simulink model "controllo_giunti_2"  (R2020b)
settings: Solver=FixedStepAuto  StartTime=0.0  StopTime=1  FixedStep=0.001  RelTol=1e-3
libraries: robotcorelib x1
(part 1 of 2)
settings Model: Creator=frasi  LastModifiedBy=frasi

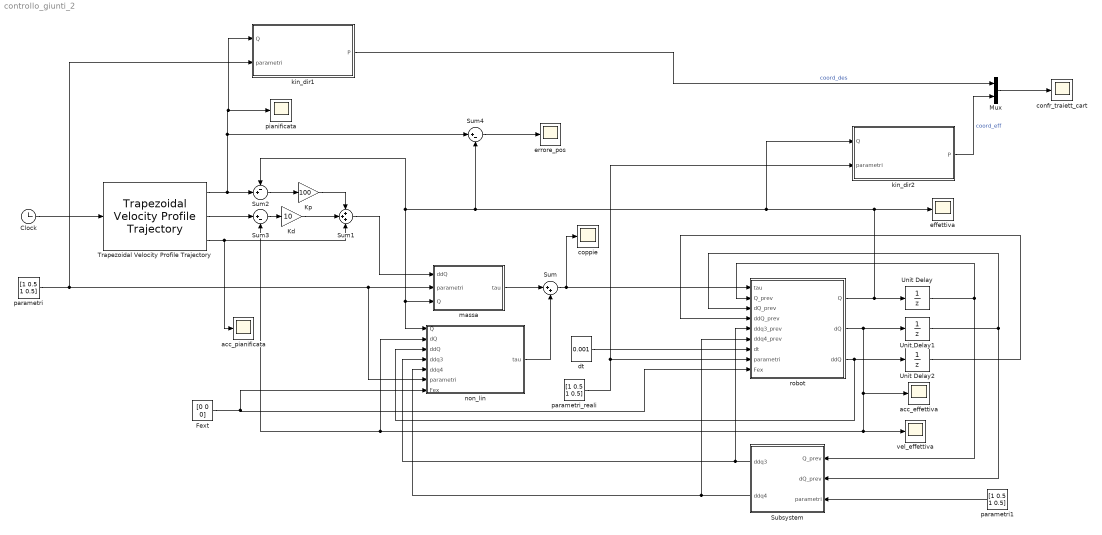
== system controllo_giunti_2 ==
  Clock : Clock
  Fext : Constant  Value=[0 0 0]
  Kd : Gain  Gain=10
  Kp : Gain  Gain=100
  Mux : Mux  Inputs=2
  Subsystem : Subsystem
  Sum : Sum  Inputs=|++
  Sum1 : Sum  Inputs=+++
  Sum2 : Sum  Inputs=-+|
  Sum3 : Sum  Inputs=|+-
  Sum4 : Sum  Inputs=|+-
  Trapezoidal Velocity Profile Trajectory : robotcorelib/Trapezoidal Velocity Profile Trajectory  WaypointSource=Internal  Waypoints=[0.5 0.7; 0.7 0.5; pi/4 pi/3]  NumParams=1  Parameter1=End Time  Parameter2=End Time  ParameterSource=Internal  PeakVelocity=[ 2; 2 ]  Acceleration=[ 1; 2 ]  EndTime=[ 1; 1 ;1]  AccelTime=[ 1; 2 ]  SimulateUsing=Interpreted execution
      settings: SourceProductBaseCode=NV,RO,RR,UV
  Unit Delay : UnitDelay  InitialCondition=[0.5 0.7 pi/4]  SampleTime=-1  HasFrameUpgradeWarning=on
  Unit Delay1 : UnitDelay  InitialCondition=[0 0 0]  SampleTime=-1  HasFrameUpgradeWarning=on
  Unit Delay2 : UnitDelay  InitialCondition=[0 0 0]  SampleTime=-1  HasFrameUpgradeWarning=on
  acc_effettiva : Scope
  acc_pianificata : Scope
  confr_traiett_cart : Scope
  coppie : Scope
  dt : Constant  Value=0.001
  effettiva : Scope
  errore_pos : Scope
  kin_dir1 : MATLAB Function  TreatAsAtomicUnit=on
  kin_dir2 : MATLAB Function  TreatAsAtomicUnit=on
  massa : MATLAB Function  TreatAsAtomicUnit=on
  non_lin : MATLAB Function  TreatAsAtomicUnit=on
  parametri : Constant  Value=[1 0.5 1 0.5]
  parametri1 : Constant  Value=[1 0.5 1 0.5]
  parametri_reali : Constant  Value=[1 0.5 1 0.5]
  pianificata : Scope
  robot : MATLAB Function  TreatAsAtomicUnit=on
  vel_effettiva : Scope
  wires:
  Clock/1 -> Trapezoidal Velocity Profile Trajectory/1
  parametri/1 -> kin_dir1/2(parametri), non_lin/6(parametri), massa/2(parametri)
  massa/1(tau) -> Sum/1
  dt/1 -> robot/7(dt)
  robot/1(Q) -> Unit Delay/1, Sum4/2, Sum2/1, massa/3(Q), non_lin/1(Q), kin_dir2/1(Q), effettiva/1
  robot/2(dQ) -> Unit Delay1/1, non_lin/2(dQ), Sum3/2, vel_effettiva/1, acc_effettiva/1
  Unit Delay/1 -> Subsystem/1(Q_prev), robot/2(Q_prev)
  Unit Delay1/1 -> Subsystem/2(dQ_prev), robot/3(dQ_prev)
  Sum/1 -> coppie/1, robot/1(tau)
  Sum1/1 -> massa/1(ddQ)
  Trapezoidal Velocity Profile Trajectory/2 -> Sum3/1
  Sum2/1 -> Kp/1
  Sum3/1 -> Kd/1
  Kp/1 -> Sum1/1
  Kd/1 -> Sum1/2
  Trapezoidal Velocity Profile Trajectory/3 -> acc_pianificata/1, Sum1/3
  non_lin/1(tau) -> Sum/2
  Trapezoidal Velocity Profile Trajectory/1 -> Sum4/1, kin_dir1/1(Q), pianificata/1, Sum2/2
  robot/3(ddQ) -> non_lin/3(ddQ), Unit Delay2/1
  parametri_reali/1 -> kin_dir2/2(parametri), robot/8(parametri)
  Sum4/1 -> errore_pos/1
  kin_dir1/1(P) -> Mux/1  "coord_des"
  kin_dir2/1(P) -> Mux/2  "coord_eff"
  Mux/1 -> confr_traiett_cart/1
  Fext/1 -> non_lin/7(Fex), robot/9(Fex)
  parametri1/1 -> Subsystem/3(parametri)
  Subsystem/2(ddq4) -> non_lin/5(ddq4), robot/6(ddq4_prev)
  Unit Delay2/1 -> robot/4(ddQ_prev)
  Subsystem/1(ddq3) -> non_lin/4(ddq3), robot/5(ddq3_prev)

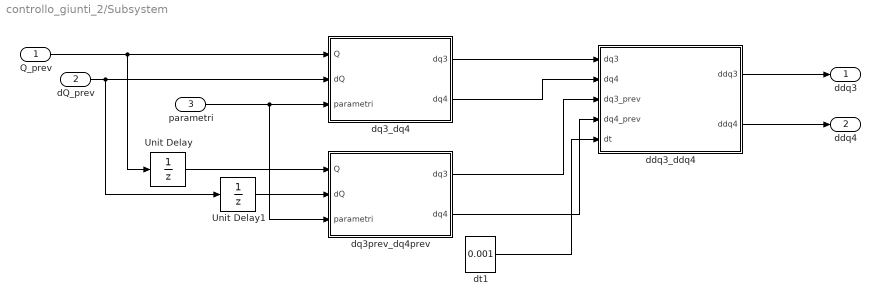
== system controllo_giunti_2/Subsystem ==
  Q_prev : Inport
  dQ_prev : Inport  Port=2
  parametri : Inport  Port=3
  Unit Delay : UnitDelay  InitialCondition=[0.5 0.7 pi/4]  SampleTime=-1  HasFrameUpgradeWarning=on
  Unit Delay1 : UnitDelay  InitialCondition=[0 0 0]  SampleTime=-1  HasFrameUpgradeWarning=on
  ddq3_ddq4 : MATLAB Function  TreatAsAtomicUnit=on
  dq3_dq4 : MATLAB Function  TreatAsAtomicUnit=on
  dq3prev_dq4prev : MATLAB Function  TreatAsAtomicUnit=on
  dt1 : Constant  Value=0.001
  ddq3 : Outport
  ddq4 : Outport  Port=2
  wires:
  ddq3_ddq4/1(ddq3) -> ddq3/1
  parametri/1 -> dq3prev_dq4prev/3(parametri), dq3_dq4/3(parametri)
  Q_prev/1 -> Unit Delay/1, dq3_dq4/1(Q)
  dq3_dq4/2(dq4) -> ddq3_ddq4/2(dq4)
  ddq3_ddq4/2(ddq4) -> ddq4/1
  dq3_dq4/1(dq3) -> ddq3_ddq4/1(dq3)
  dt1/1 -> ddq3_ddq4/5(dt)
  dq3prev_dq4prev/1(dq3) -> ddq3_ddq4/3(dq3_prev)
  dq3prev_dq4prev/2(dq4) -> ddq3_ddq4/4(dq4_prev)
  dQ_prev/1 -> Unit Delay1/1, dq3_dq4/2(dQ)
  Unit Delay1/1 -> dq3prev_dq4prev/2(dQ)
  Unit Delay/1 -> dq3prev_dq4prev/1(Q)

== matlab function controllo_giunti_2/non_lin ==
  data: Q input; tau output; dQ input; ddQ input; ddq3 input; ddq4 input; parametri input; Fex input
function tau = non_lin(Q,dQ,ddQ,ddq3,ddq4,parametri,Fex)
l=parametri(1);
d=parametri(2);
m1=parametri(3);
ma=parametri(4);

xc1=Q(1);
xc5=Q(2);
q2=Q(3);

dxc1=dQ(1);
dxc5=dQ(2);
dq2=dQ(3);

ddxc1=ddQ(1);
ddxc5=ddQ(2);
ddq2=ddQ(3);

Fx=Fex(1);
Fy=Fex(2);
Mf=Fex(3);

I2 = ma*l^2/4 + 1/12 *ma*l^2;
I5 = I2;
I3 = I2 + 1/12 * ma*d^2 + ma*(d^2/4+l^2/4);

q3 = ...
 -q2 - 2*atan((2*l*xc5 + (-(2*l*xc1 + l^2 + l^2*tan(q2/2)^2 + xc1^2 + xc5^2 + xc1^2*tan(q2/2)^2 + xc5^2*tan(q2/2)^2 - 4*l*xc5*tan(q2/2) - 2*l*xc1*tan(q2/2)^2)*(2*l*xc1 - 3*l^2 - 3*l^2*tan(q2/2)^2 + xc1^2 + xc5^2 + xc1^2*tan(q2/2)^2 + xc5^2*tan(q2/2)^2 - 4*l*xc5*tan(q2/2) - 2*l*xc1*tan(q2/2)^2))^(1/2) - 4*l^2*tan(q2/2) + 2*l*xc5*tan(q2/2)^2)/(3*l^2*tan(q2/2)^2 - l^2 + xc1^2 + xc5^2 + xc1^2*tan(q2/2)^2 + xc5^2*tan(q2/2)^2 - 4*l*xc5*tan(q2/2) - 4*l*xc1*tan(q2/2)^2) - (4*(l*xc5 - 2*l^2*tan(q2/2) + l*xc5*tan(q2/2)^2))/(3*l^2*tan(q2/2)^2 - l^2 + xc1^2 + xc5^2 + xc1^2*tan(q2/2)^2 + xc5^2*tan(q2/2)^2 - 4*l*xc5*tan(q2/2) - 4*l*xc1*tan(q2/2)^2));
q4 = ...
2*atan((2*l*xc5 + (-(2*l*xc1 + l^2 + l^2*tan(q2/2)^2 + xc1^2 + xc5^2 + xc1^2*tan(q2/2)^2 + xc5^2*tan(q2/2)^2 - 4*l*xc5*tan(q2/2) - 2*l*xc1*tan(q2/2)^2)*(2*l*xc1 - 3*l^2 - 3*l^2*tan(q2/2)^2 + xc1^2 + xc5^2 + xc1^2*tan(q2/2)^2 + xc5^2*tan(q2/2)^2 - 4*l*xc5*tan(q2/2) - 2*l*xc1*tan(q2/2)^2))^(1/2) - 4*l^2*tan(q2/2) + 2*l*xc5*tan(q2/2)^2)/(3*l^2*tan(q2/2)^2 - l^2 + xc1^2 + xc5^2 + xc1^2*tan(q2/2)^2 + xc5^2*tan(q2/2)^2 - 4*l*xc5*tan(q2/2) - 4*l*xc1*tan(q2/2)^2)) + 2*atan((2*l*xc5 + (-(2*l*xc1 + l^2 + l^2*tan(q2/2)^2 + xc1^2 + xc5^2 + xc1^2*tan(q2/2)^2 + xc5^2*tan(q2/2)^2 - 4*l*xc5*tan(q2/2) - 2*l*xc1*tan(q2/2)^2)*(2*l*xc1 - 3*l^2 - 3*l^2*tan(q2/2)^2 + xc1^2 + xc5^2 + xc1^2*tan(q2/2)^2 + xc5^2*tan(q2/2)^2 - 4*l*xc5*tan(q2/2) - 2*l*xc1*tan(q2/2)^2))^(1/2) - 4*l^2*tan(q2/2) + 2*l*xc5*tan(q2/2)^2)/(3*l^2*tan(q2/2)^2 - l^2 + xc1^2 + xc5^2 + xc1^2*tan(q2/2)^2 + xc5^2*tan(q2/2)^2 - 4*l*xc5*tan(q2/2) - 4*l*xc1*tan(q2/2)^2) - (4*(l*xc5 - 2*l^2*tan(q2/2) + l*xc5*tan(q2/2)^2))/(3*l^2*tan(q2/2)^2 - l^2 + xc1^2 + xc5^2 + xc1^2*tan(q2/2)^2 + xc5^2*tan(q2/2)^2 - 4*l*xc5*tan(q2/2) - 4*l*xc1*tan(q2/2)^2));

dq3 =...
(2*dxc5*((2*l + (4*sin(q2)*l^3 - 4*sin(2*q2)*l^2*xc1 - 4*cos(2*q2)*l^2*xc5 - 4*sin(q2)*l*xc1^2 + 8*cos(q2)*l*xc1*xc5 - 12*sin(q2)*l*xc5^2 + 4*xc1^2*xc5 + 4*xc5^3)/(2*(3*l^4 + 4*cos(q2)*l^3*xc1 - 4*sin(q2)*l^3*xc5 - 2*cos(2*q2)*l^2*xc1^2 + 4*sin(2*q2)*l^2*xc1*xc5 + 2*cos(2*q2)*l^2*xc5^2 - 4*cos(q2)*l*xc1^3 + 4*sin(q2)*l*xc1^2*xc5 - 4*cos(q2)*l*xc1*xc5^2 + 4*sin(q2)*l*xc5^3 - xc1^4 - 2*xc1^2*xc5^2 - xc5^4)^(1/2)))/(l^2 - 2*l*xc1 + xc1^2 + xc5^2 - 2*l^2*cos(q2) + 2*l*xc1*cos(q2) - 2*l*xc5*sin(q2)) + ((2*xc5 - 2*l*sin(q2))*(2*l^2*sin(q2) + (3*l^4 + 4*cos(q2)*l^3*xc1 - 4*sin(q2)*l^3*xc5 - 2*cos(2*q2)*l^2*xc1^2 + 4*sin(2*q2)*l^2*xc1*xc5 + 2*cos(2*q2)*l^2*xc5^2 - 4*cos(q2)*l*xc1^3 + 4*sin(q2)*l*xc1^2*xc5 - 4*cos(q2)*l*xc1*xc5^2 + 4*sin(q2)*l*xc5^3 - xc1^4 - 2*xc1^2*xc5^2 - xc5^4)^(1/2) - 2*l*xc5))/(l^2 - 2*l*xc1 + xc1^2 + xc5^2 - 2*l^2*cos(q2) + 2*l*xc1*cos(q2) - 2*l*xc5*sin(q2))^2))/((2*l^2*sin(q2) + (3*l^4 + 4*cos(q2)*l^3*xc1 - 4*sin(q2)*l^3*xc5 - 2*cos(2*q2)*l^2*xc1^2 + 4*sin(2*q2)*l^2*xc1*xc5 + 2*cos(2*q2)*l^2*xc5^2 - 4*cos(q2)*l*xc1^3 + 4*sin(q2)*l*xc1^2*xc5 - 4*cos(q2)*l*xc1*xc5^2 + 4*sin(q2)*l*xc5^3 - xc1^4 - 2*xc1^2*xc5^2 - xc5^4)^(1/2) - 2*l*xc5)^2/(l^2 - 2*l*xc1 + xc1^2 + xc5^2 - 2*l^2*cos(q2) + 2*l*xc1*cos(q2) - 2*l*xc5*sin(q2))^2 + 1) - dq2*((2*(((- 4*sin(q2)*l^3*xc1 - 4*cos(q2)*l^3*xc5 + 4*sin(2*q2)*l^2*xc1^2 + 8*cos(2*q2)*l^2*xc1*xc5 - 4*sin(2*q2)*l^2*xc5^2 + 4*sin(q2)*l*xc1^3 + 4*cos(q2)*l*xc1^2*xc5 + 4*sin(q2)*l*xc1*xc5^2 + 4*cos(q2)*l*xc5^3)/(2*(3*l^4 + 4*cos(q2)*l^3*xc1 - 4*sin(q2)*l^3*xc5 - 2*cos(2*q2)*l^2*xc1^2 + 4*sin(2*q2)*l^2*xc1*xc5 + 2*cos(2*q2)*l^2*xc5^2 - 4*cos(q2)*l*xc1^3 + 4*sin(q2)*l*xc1^2*xc5 - 4*cos(q2)*l*xc1*xc5^2 + 4*sin(q2)*l*xc5^3 - xc1^4 - 2*xc1^2*xc5^2 - xc5^4)^(1/2)) + 2*l^2*cos(q2))/(l^2 - 2*l*xc1 + xc1^2 + xc5^2 - 2*l^2*cos(q2) + 2*l*xc1*cos(q2) - 2*l*xc5*sin(q2)) + ((2*l*xc5*cos(q2) - 2*l^2*sin(q2) + 2*l*xc1*sin(q2))*(2*l^2*sin(q2) + (3*l^4 + 4*cos(q2)*l^3*xc1 - 4*sin(q2)*l^3*xc5 - 2*cos(2*q2)*l^2*xc1^2 + 4*sin(2*q2)*l^2*xc1*xc5 + 2*cos(2*q2)*l^2*xc5^2 - 4*cos(q2)*l*xc1^3 + 4*sin(q2)*l*xc1^2*xc5 - 4*cos(q2)*l*xc1*xc5^2 + 4*sin(q2)*l*xc5^3 - xc1^4 - 2*xc1^2*xc5^2 - xc5^4)^(1/2) - 2*l*xc5))/(l^2 - 2*l*xc1 + xc1^2 + xc5^2 - 2*l^2*cos(q2) + 2*l*xc1*cos(q2) - 2*l*xc5*sin(q2))^2))/((2*l^2*sin(q2) + (3*l^4 + 4*cos(q2)*l^3*xc1 - 4*sin(q2)*l^3*xc5 - 2*cos(2*q2)*l^2*xc1^2 + 4*sin(2*q2)*l^2*xc1*xc5 + 2*cos(2*q2)*l^2*xc5^2 - 4*cos(q2)*l*xc1^3 + 4*sin(q2)*l*xc1^2*xc5 - 4*cos(q2)*l*xc1*xc5^2 + 4*sin(q2)*l*xc5^3 - xc1^4 - 2*xc1^2*xc5^2 - xc5^4)^(1/2) - 2*l*xc5)^2/(l^2 - 2*l*xc1 + xc1^2 + xc5^2 - 2*l^2*cos(q2) + 2*l*xc1*cos(q2) - 2*l*xc5*sin(q2))^2 + 1) + 1) + (2*dxc1*(((2*xc1 - 2*l + 2*l*cos(q2))*(2*l^2*sin(q2) + (3*l^4 + 4*cos(q2)*l^3*xc1 - 4*sin(q2)*l^3*xc5 - 2*cos(2*q2)*l^2*xc1^2 + 4*sin(2*q2)*l^2*xc1*xc5 + 2*cos(2*q2)*l^2*xc5^2 - 4*cos(q2)*l*xc1^3 + 4*sin(q2)*l*xc1^2*xc5 - 4*cos(q2)*l*xc1*xc5^2 + 4*sin(q2)*l*xc5^3 - xc1^4 - 2*xc1^2*xc5^2 - xc5^4)^(1/2) - 2*l*xc5))/(l^2 - 2*l*xc1 + xc1^2 + xc5^2 - 2*l^2*cos(q2) + 2*l*xc1*cos(q2) - 2*l*xc5*sin(q2))^2 + (- 4*cos(q2)*l^3 + 4*cos(2*q2)*l^2*xc1 - 4*sin(2*q2)*l^2*xc5 + 12*cos(q2)*l*xc1^2 - 8*sin(q2)*l*xc1*xc5 + 4*cos(q2)*l*xc5^2 + 4*xc1^3 + 4*xc1*xc5^2)/(2*(l^2 - 2*l*xc1 + xc1^2 + xc5^2 - 2*l^2*cos(q2) + 2*l*xc1*cos(q2) - 2*l*xc5*sin(q2))*(3*l^4 + 4*cos(q2)*l^3*xc1 - 4*sin(q2)*l^3*xc5 - 2*cos(2*q2)*l^2*xc1^2 + 4*sin(2*q2)*l^2*xc1*xc5 + 2*cos(2*q2)*l^2*xc5^2 - 4*cos(q2)*l*xc1^3 + 4*sin(q2)*l*xc1^2*xc5 - 4*cos(q2)*l*xc1*xc5^2 + 4*sin(q2)*l*xc5^3 - xc1^4 - 2*xc1^2*xc5^2 - xc5^4)^(1/2))))/((2*l^2*sin(q2) + (3*l^4 + 4*cos(q2)*l^3*xc1 - 4*sin(q2)*l^3*xc5 - 2*cos(2*q2)*l^2*xc1^2 + 4*sin(2*q2)*l^2*xc1*xc5 + 2*cos(2*q2)*l^2*xc5^2 - 4*cos(q2)*l*xc1^3 + 4*sin(q2)*l*xc1^2*xc5 - 4*cos(q2)*l*xc1*xc5^2 + 4*sin(q2)*l*xc5^3 - xc1^4 - 2*xc1^2*xc5^2 - xc5^4)^(1/2) - 2*l*xc5)^2/(l^2 - 2*l*xc1 + xc1^2 + xc5^2 - 2*l^2*cos(q2) + 2*l*xc1*cos(q2) - 2*l*xc5*sin(q2))^2 + 1);

dq4 =...
 - dxc1*((2*(((2*xc1 - 2*l + 2*l*cos(q2))*((3*l^4 + 4*cos(q2)*l^3*xc1 - 4*sin(q2)*l^3*xc5 - 2*cos(2*q2)*l^2*xc1^2 + 4*sin(2*q2)*l^2*xc1*xc5 + 2*cos(2*q2)*l^2*xc5^2 - 4*cos(q2)*l*xc1^3 + 4*sin(q2)*l*xc1^2*xc5 - 4*cos(q2)*l*xc1*xc5^2 + 4*sin(q2)*l*xc5^3 - xc1^4 - 2*xc1^2*xc5^2 - xc5^4)^(1/2) - 2*l^2*sin(q2) + 2*l*xc5))/(l^2 - 2*l*xc1 + xc1^2 + xc5^2 - 2*l^2*cos(q2) + 2*l*xc1*cos(q2) - 2*l*xc5*sin(q2))^2 + (2*(xc1 + l*cos(q2))*(- l^2 + 2*cos(q2)*l*xc1 - 2*sin(q2)*l*xc5 + xc1^2 + xc5^2))/((l^2 - 2*l*xc1 + xc1^2 + xc5^2 - 2*l^2*cos(q2) + 2*l*xc1*cos(q2) - 2*l*xc5*sin(q2))*(3*l^4 + 4*cos(q2)*l^3*xc1 - 4*sin(q2)*l^3*xc5 - 2*cos(2*q2)*l^2*xc1^2 + 4*sin(2*q2)*l^2*xc1*xc5 + 2*cos(2*q2)*l^2*xc5^2 - 4*cos(q2)*l*xc1^3 + 4*sin(q2)*l*xc1^2*xc5 - 4*cos(q2)*l*xc1*xc5^2 + 4*sin(q2)*l*xc5^3 - xc1^4 - 2*xc1^2*xc5^2 - xc5^4)^(1/2))))/(((3*l^4 + 4*cos(q2)*l^3*xc1 - 4*sin(q2)*l^3*xc5 - 2*cos(2*q2)*l^2*xc1^2 + 4*sin(2*q2)*l^2*xc1*xc5 + 2*cos(2*q2)*l^2*xc5^2 - 4*cos(q2)*l*xc1^3 + 4*sin(q2)*l*xc1^2*xc5 - 4*cos(q2)*l*xc1*xc5^2 + 4*sin(q2)*l*xc5^3 - xc1^4 - 2*xc1^2*xc5^2 - xc5^4)^(1/2) - 2*l^2*sin(q2) + 2*l*xc5)^2/(l^2 - 2*l*xc1 + xc1^2 + xc5^2 - 2*l^2*cos(q2) + 2*l*xc1*cos(q2) - 2*l*xc5*sin(q2))^2 + 1) + (2*(((2*xc1 - 2*l + 2*l*cos(q2))*(2*l^2*sin(q2) + (3*l^4 + 4*cos(q2)*l^3*xc1 - 4*sin(q2)*l^3*xc5 - 2*cos(2*q2)*l^2*xc1^2 + 4*sin(2*q2)*l^2*xc1*xc5 + 2*cos(2*q2)*l^2*xc5^2 - 4*cos(q2)*l*xc1^3 + 4*sin(q2)*l*xc1^2*xc5 - 4*cos(q2)*l*xc1*xc5^2 + 4*sin(q2)*l*xc5^3 - xc1^4 - 2*xc1^2*xc5^2 - xc5^4)^(1/2) - 2*l*xc5))/(l^2 - 2*l*xc1 + xc1^2 + xc5^2 - 2*l^2*cos(q2) + 2*l*xc1*cos(q2) - 2*l*xc5*sin(q2))^2 + (2*(xc1 + l*cos(q2))*(- l^2 + 2*cos(q2)*l*xc1 - 2*sin(q2)*l*xc5 + xc1^2 + xc5^2))/((l^2 - 2*l*xc1 + xc1^2 + xc5^2 - 2*l^2*cos(q2) + 2*l*xc1*cos(q2) - 2*l*xc5*sin(q2))*(3*l^4 + 4*cos(q2)*l^3*xc1 - 4*sin(q2)*l^3*xc5 - 2*cos(2*q2)*l^2*xc1^2 + 4*sin(2*q2)*l^2*xc1*xc5 + 2*cos(2*q2)*l^2*xc5^2 - 4*cos(q2)*l*xc1^3 + 4*sin(q2)*l*xc1^2*xc5 - 4*cos(q2)*l*xc1*xc5^2 + 4*sin(q2)*l*xc5^3 - xc1^4 - 2*xc1^2*xc5^2 - xc5^4)^(1/2))))/((2*l^2*sin(q2) + (3*l^4 + 4*cos(q2)*l^3*xc1 - 4*sin(q2)*l^3*xc5 - 2*cos(2*q2)*l^2*xc1^2 + 4*sin(2*q2)*l^2*xc1*xc5 + 2*cos(2*q2)*l^2*xc5^2 - 4*cos(q2)*l*xc1^3 + 4*sin(q2)*l*xc1^2*xc5 - 4*cos(q2)*l*xc1*xc5^2 + 4*sin(q2)*l*xc5^3 - xc1^4 - 2*xc1^2*xc5^2 - xc5^4)^(1/2) - 2*l*xc5)^2/(l^2 - 2*l*xc1 + xc1^2 + xc5^2 - 2*l^2*cos(q2) + 2*l*xc1*cos(q2) - 2*l*xc5*sin(q2))^2 + 1)) - dxc5*((2*((2*l + (2*sin(q2)*l^3 - 2*sin(2*q2)*l^2*xc1 - 2*cos(2*q2)*l^2*xc5 - 2*sin(q2)*l*xc1^2 + 4*cos(q2)*l*xc1*xc5 - 6*sin(q2)*l*xc5^2 + 2*xc1^2*xc5 + 2*xc5^3)/(3*l^4 + 4*cos(q2)*l^3*xc1 - 4*sin(q2)*l^3*xc5 - 2*cos(2*q2)*l^2*xc1^2 + 4*sin(2*q2)*l^2*xc1*xc5 + 2*cos(2*q2)*l^2*xc5^2 - 4*cos(q2)*l*xc1^3 + 4*sin(q2)*l*xc1^2*xc5 - 4*cos(q2)*l*xc1*xc5^2 + 4*sin(q2)*l*xc5^3 - xc1^4 - 2*xc1^2*xc5^2 - xc5^4)^(1/2))/(l^2 - 2*l*xc1 + xc1^2 + xc5^2 - 2*l^2*cos(q2) + 2*l*xc1*cos(q2) - 2*l*xc5*sin(q2)) + ((2*xc5 - 2*l*sin(q2))*(2*l^2*sin(q2) + (3*l^4 + 4*cos(q2)*l^3*xc1 - 4*sin(q2)*l^3*xc5 - 2*cos(2*q2)*l^2*xc1^2 + 4*sin(2*q2)*l^2*xc1*xc5 + 2*cos(2*q2)*l^2*xc5^2 - 4*cos(q2)*l*xc1^3 + 4*sin(q2)*l*xc1^2*xc5 - 4*cos(q2)*l*xc1*xc5^2 + 4*sin(q2)*l*xc5^3 - xc1^4 - 2*xc1^2*xc5^2 - xc5^4)^(1/2) - 2*l*xc5))/(l^2 - 2*l*xc1 + xc1^2 + xc5^2 - 2*l^2*cos(q2) + 2*l*xc1*cos(q2) - 2*l*xc5*sin(q2))^2))/((2*l^2*sin(q2) + (3*l^4 + 4*cos(q2)*l^3*xc1 - 4*sin(q2)*l^3*xc5 - 2*cos(2*q2)*l^2*xc1^2 + 4*sin(2*q2)*l^2*xc1*xc5 + 2*cos(2*q2)*l^2*xc5^2 - 4*cos(q2)*l*xc1^3 + 4*sin(q2)*l*xc1^2*xc5 - 4*cos(q2)*l*xc1*xc5^2 + 4*sin(q2)*l*xc5^3 - xc1^4 - 2*xc1^2*xc5^2 - xc5^4)^(1/2) - 2*l*xc5)^2/(l^2 - 2*l*xc1 + xc1^2 + xc5^2 - 2*l^2*cos(q2) + 2*l*xc1*cos(q2) - 2*l*xc5*sin(q2))^2 + 1) - (2*((2*l - (2*sin(q2)*l^3 - 2*sin(2*q2)*l^2*xc1 - 2*cos(2*q2)*l^2*xc5 - 2*sin(q2)*l*xc1^2 + 4*cos(q2)*l*xc1*xc5 - 6*sin(q2)*l*xc5^2 + 2*xc1^2*xc5 + 2*xc5^3)/(3*l^4 + 4*cos(q2)*l^3*xc1 - 4*sin(q2)*l^3*xc5 - 2*cos(2*q2)*l^2*xc1^2 + 4*sin(2*q2)*l^2*xc1*xc5 + 2*cos(2*q2)*l^2*xc5^2 - 4*cos(q2)*l*xc1^3 + 4*sin(q2)*l*xc1^2*xc5 - 4*cos(q2)*l*xc1*xc5^2 + 4*sin(q2)*l*xc5^3 - xc1^4 - 2*xc1^2*xc5^2 - xc5^4)^(1/2))/(l^2 - 2*l*xc1 + xc1^2 + xc5^2 - 2*l^2*cos(q2) + 2*l*xc1*cos(q2) - 2*l*xc5*sin(q2)) - ((2*xc5 - 2*l*sin(q2))*((3*l^4 + 4*cos(q2)*l^3*xc1 - 4*sin(q2)*l^3*xc5 - 2*cos(2*q2)*l^2*xc1^2 + 4*sin(2*q2)*l^2*xc1*xc5 + 2*cos(2*q2)*l^2*xc5^2 - 4*cos(q2)*l*xc1^3 + 4*sin(q2)*l*xc1^2*xc5 - 4*cos(q2)*l*xc1*xc5^2 + 4*sin(q2)*l*xc5^3 - xc1^4 - 2*xc1^2*xc5^2 - xc5^4)^(1/2) - 2*l^2*sin(q2) + 2*l*xc5))/(l^2 - 2*l*xc1 + xc1^2 + xc5^2 - 2*l^2*cos(q2) + 2*l*xc1*cos(q2) - 2*l*xc5*sin(q2))^2))/(((3*l^4 + 4*cos(q2)*l^3*xc1 - 4*sin(q2)*l^3*xc5 - 2*cos(2*q2)*l^2*xc1^2 + 4*sin(2*q2)*l^2*xc1*xc5 + 2*cos(2*q2)*l^2*xc5^2 - 4*cos(q2)*l*xc1^3 + 4*sin(q2)*l*xc1^2*xc5 - 4*cos(q2)*l*xc1*xc5^2 + 4*sin(q2)*l*xc5^3 - xc1^4 - 2*xc1^2*xc5^2 - xc5^4)^(1/2) - 2*l^2*sin(q2) + 2*l*xc5)^2/(l^2 - 2*l*xc1 + xc1^2 + xc5^2 - 2*l^2*cos(q2) + 2*l*xc1*cos(q2) - 2*l*xc5*sin(q2))^2 + 1)) - dq2*((2*((2*l^2*cos(q2) - (2*l*(- sin(q2)*l^2*xc1 - cos(q2)*l^2*xc5 + sin(2*q2)*l*xc1^2 + 2*cos(2*q2)*l*xc1*xc5 - sin(2*q2)*l*xc5^2 + sin(q2)*xc1^3 + cos(q2)*xc1^2*xc5 + sin(q2)*xc1*xc5^2 + cos(q2)*xc5^3))/(3*l^4 + 4*cos(q2)*l^3*xc1 - 4*sin(q2)*l^3*xc5 - 2*cos(2*q2)*l^2*xc1^2 + 4*sin(2*q2)*l^2*xc1*xc5 + 2*cos(2*q2)*l^2*xc5^2 - 4*cos(q2)*l*xc1^3 + 4*sin(q2)*l*xc1^2*xc5 - 4*cos(q2)*l*xc1*xc5^2 + 4*sin(q2)*l*xc5^3 - xc1^4 - 2*xc1^2*xc5^2 - xc5^4)^(1/2))/(l^2 - 2*l*xc1 + xc1^2 + xc5^2 - 2*l^2*cos(q2) + 2*l*xc1*cos(q2) - 2*l*xc5*sin(q2)) - (2*l*(xc5*cos(q2) - l*sin(q2) + xc1*sin(q2))*((3*l^4 + 4*cos(q2)*l^3*xc1 - 4*sin(q2)*l^3*xc5 - 2*cos(2*q2)*l^2*xc1^2 + 4*sin(2*q2)*l^2*xc1*xc5 + 2*cos(2*q2)*l^2*xc5^2 - 4*cos(q2)*l*xc1^3 + 4*sin(q2)*l*xc1^2*xc5 - 4*cos(q2)*l*xc1*xc5^2 + 4*sin(q2)*l*xc5^3 - xc1^4 - 2*xc1^2*xc5^2 - xc5^4)^(1/2) - 2*l^2*sin(q2) + 2*l*xc5))/(l^2 - 2*l*xc1 + xc1^2 + xc5^2 - 2*l^2*cos(q2) + 2*l*xc1*cos(q2) - 2*l*xc5*sin(q2))^2))/(((3*l^4 + 4*cos(q2)*l^3*xc1 - 4*sin(q2)*l^3*xc5 - 2*cos(2*q2)*l^2*xc1^2 + 4*sin(2*q2)*l^2*xc1*xc5 + 2*cos(2*q2)*l^2*xc5^2 - 4*cos(q2)*l*xc1^3 + 4*sin(q2)*l*xc1^2*xc5 - 4*cos(q2)*l*xc1*xc5^2 + 4*sin(q2)*l*xc5^3 - xc1^4 - 2*xc1^2*xc5^2 - xc5^4)^(1/2) - 2*l^2*sin(q2) + 2*l*xc5)^2/(l^2 - 2*l*xc1 + xc1^2 + xc5^2 - 2*l^2*cos(q2) + 2*l*xc1*cos(q2) - 2*l*xc5*sin(q2))^2 + 1) - (2*((2*l^2*cos(q2) + (2*l*(- sin(q2)*l^2*xc1 - cos(q2)*l^2*xc5 + sin(2*q2)*l*xc1^2 + 2*cos(2*q2)*l*xc1*xc5 - sin(2*q2)*l*xc5^2 + sin(q2)*xc1^3 + cos(q2)*xc1^2*xc5 + sin(q2)*xc1*xc5^2 + cos(q2)*xc5^3))/(3*l^4 + 4*cos(q2)*l^3*xc1 - 4*sin(q2)*l^3*xc5 - 2*cos(2*q2)*l^2*xc1^2 + 4*sin(2*q2)*l^2*xc1*xc5 + 2*cos(2*q2)*l^2*xc5^2 - 4*cos(q2)*l*xc1^3 + 4*sin(q2)*l*xc1^2*xc5 - 4*cos(q2)*l*xc1*xc5^2 + 4*sin(q2)*l*xc5^3 - xc1^4 - 2*xc1^2*xc5^2 - xc5^4)^(1/2))/(l^2 - 2*l*xc1 + xc1^2 + xc5^2 - 2*l^2*cos(q2) + 2*l*xc1*cos(q2) - 2*l*xc5*sin(q2)) + (2*l*(xc5*cos(q2) - l*sin(q2) + xc1*sin(q2))*(2*l^2*sin(q2) + (3*l^4 + 4*cos(q2)*l^3*xc1 - 4*sin(q2)*l^3*xc5 - 2*cos(2*q2)*l^2*xc1^2 + 4*sin(2*q2)*l^2*xc1*xc5 + 2*cos(2*q2)*l^2*xc5^2 - 4*cos(q2)*l*xc1^3 + 4*sin(q2)*l*xc1^2*xc5 - 4*cos(q2)*l*xc1*xc5^2 + 4*sin(q2)*l*xc5^3 - xc1^4 - 2*xc1^2*xc5^2 - xc5^4)^(1/2) - 2*l*xc5))/(l^2 - 2*l*xc1 + xc1^2 + xc5^2 - 2*l^2*cos(q2) + 2*l*xc1*cos(q2) - 2*l*xc5*sin(q2))^2))/((2*l^2*sin(q2) + (3*l^4 + 4*cos(q2)*l^3*xc1 - 4*sin(q2)*l^3*xc5 - 2*cos(2*q2)*l^2*xc1^2 + 4*sin(2*q2)*l^2*xc1*xc5 + 2*cos(2*q2)*l^2*xc5^2 - 4*cos(q2)*l*xc1^3 + 4*sin(q2)*l*xc1^2*xc5 - 4*cos(q2)*l*xc1*xc5^2 + 4*sin(q2)*l*xc5^3 - xc1^4 - 2*xc1^2*xc5^2 - xc5^4)^(1/2) - 2*l*xc5)^2/(l^2 - 2*l*xc1 + xc1^2 + xc5^2 - 2*l^2*cos(q2) + 2*l*xc1*cos(q2) - 2*l*xc5*sin(q2))^2 + 1));

ddx2=ddxc1-l/2*(cos(q2)*dq2^2+sin(q2)*ddq2);
q5=q2+q3+q4-pi;
dq5=dq2+dq3+dq4;
ddq5=ddq2+ddq3+ddq4;
ddy4=ddxc5+ddq5*l/2*cos(q5)-dq5^2*l/2*sin(q5);

g=9.81;

G=...
[                  -(ma*(3*l*cos(q4) + 3*l*cos(2*q2 + 2*q3 + q4) - d*sin(q4) + d*sin(2*q2 + 2*q3 + q4)))/(4*l*sin(q4));...
(d*ma*cos(q4) - d*ma*cos(2*q2 + 2*q3 + q4) + 4*l*m1*sin(q4) + 5*l*ma*sin(q4) + 3*l*ma*sin(2*q2 + 2*q3 + q4))/(4*l*sin(q4));...
-(ma*(3*l*sin(q2 + 2*q3 + q4) - d*cos(q2 + 2*q3 + q4) - 6*l*sin(q2 + q4) + d*cos(q2 - q4) + 3*l*sin(q2 - q4)))/(4*sin(q4))];

V=...
   [(4*Mf*cos(q2 + q3 + q4) + 3*l*ma*cos(q4) + 3*l*ma*cos(2*q2 + 2*q3 + q4) - d*ma*sin(q4) + d*ma*sin(2*q2 + 2*q3 + q4) - 4*I3*ddq3*cos(q2 + q3 + q4) + 4*I5*ddq3*cos(q2 + q3) + 4*I5*ddq4*cos(q2 + q3) - 4*Fx*l*sin(q4) - 4*dq2^2*l^2*ma*sin(q2 + q4) + 2*ddq3*l^2*ma*cos(q2 + q3 + q4) + 4*dq2^2*l^2*ma*sin(q2 - q4) - 2*ddq3*l^2*ma*cos(q2 + q3 - q4) - 3*g*l*ma*cos(q4) - 3*g*l*ma*cos(2*q2 + 2*q3 + q4) + d*g*ma*sin(q4) - d*g*ma*sin(2*q2 + 2*q3 + q4) + 4*ddx2*l*ma*sin(q4) - 2*dq2^2*l^2*ma*sin(q2 + q3 + q4) - 2*dq3^2*l^2*ma*sin(q2 + q3 + q4) + 2*dq2^2*l^2*ma*sin(q2 + q3 - q4) + 2*dq3^2*l^2*ma*sin(q2 + q3 - q4) + 4*d*ddq3*l*ma*sin(q2 + q3 + q4) + 4*d*dq2^2*l*ma*cos(q2 + q3 + q4) + 4*d*dq3^2*l*ma*cos(q2 + q3 + q4) - 4*d*ddq3*l*ma*sin(q2 + q3 - q4) - 4*dq2*dq3*l^2*ma*sin(q2 + q3 + q4) - 4*d*dq2^2*l*ma*cos(q2 + q3 - q4) - 4*d*dq3^2*l*ma*cos(q2 + q3 - q4) + 4*dq2*dq3*l^2*ma*sin(q2 + q3 - q4) + 8*d*dq2*dq3*l*ma*cos(q2 + q3 + q4) - 8*d*dq2*dq3*l*ma*cos(q2 + q3 - q4))/(4*l*sin(q4));...
                                                                                                                                                                                                                                                                                                                                                                                                                                                                                                                                                                                                                            -(4*Mf*sin(q2 + q3 + q4) + d*ma*cos(q4) - d*ma*cos(2*q2 + 2*q3 + q4) + 4*l*m1*sin(q4) + 5*l*ma*sin(q4) + 3*l*ma*sin(2*q2 + 2*q3 + q4) - 4*I3*ddq3*sin(q2 + q3 + q4) + 4*I5*ddq3*sin(q2 + q3) + 4*I5*ddq4*sin(q2 + q3) - d*g*ma*cos(q4) + d*g*ma*cos(2*q2 + 2*q3 + q4) - 4*ddy4*l*ma*sin(q4) - 4*g*l*m1*sin(q4) - 5*g*l*ma*sin(q4) - 3*g*l*ma*sin(2*q2 + 2*q3 + q4))/(4*l*sin(q4));...
                                                       (4*Mf*sin(q3 + q4) + 2*Fx*l*cos(q2 - q4) + 2*Fy*l*sin(q2 - q4) + d*ma*cos(q2 - q4) + 3*l*ma*sin(q2 - q4) - d*ma*cos(q2 + 2*q3 + q4) - 2*Fx*l*cos(q2 + q4) + 3*l*ma*sin(q2 + 2*q3 + q4) - 4*I3*ddq3*sin(q3 + q4) - 2*Fy*l*sin(q2 + q4) - 6*l*ma*sin(q2 + q4) + 4*I5*ddq3*sin(q3) + 4*I5*ddq4*sin(q3) + 2*dq2^2*l^2*ma*cos(q3 + q4) + 2*dq3^2*l^2*ma*cos(q3 + q4) + d*g*ma*cos(q2 + 2*q3 + q4) - 2*ddq3*l^2*ma*sin(q3 - q4) - 3*g*l*ma*sin(q2 + 2*q3 + q4) + 6*g*l*ma*sin(q2 + q4) - 2*dq2^2*l^2*ma*cos(q3 - q4) - 2*dq3^2*l^2*ma*cos(q3 - q4) - d*g*ma*cos(q2 - q4) + 2*ddq3*l^2*ma*sin(q3 + q4) - 3*g*l*ma*sin(q2 - q4) + 4*d*ddq3*l*ma*cos(q3 - q4) + 4*dq2*dq3*l^2*ma*cos(q3 + q4) + 4*d*dq2^2*l*ma*sin(q3 + q4) + 4*d*dq3^2*l*ma*sin(q3 + q4) - 4*dq2*dq3*l^2*ma*cos(q3 - q4) - 4*d*dq2^2*l*ma*sin(q3 - q4) - 4*d*dq3^2*l*ma*sin(q3 - q4) - 4*d*ddq3*l*ma*cos(q3 + q4) + 8*d*dq2*dq3*l*ma*sin(q3 + q4) - 8*d*dq2*dq3*l*ma*sin(q3 - q4))/(4*sin(q4))];
N=G+V;

tau=N;
end

== matlab function controllo_giunti_2/massa ==
  data: ddQ input; parametri input; tau output; Q input
function tau = massa(ddQ,parametri,Q)
l=parametri(1);
d=parametri(2);
m1=parametri(3);
ma=parametri(4);

xc1=Q(1);
xc5=Q(2);
q2=Q(3);

q3 = ...
 -q2 - 2*atan((2*l*xc5 + (-(2*l*xc1 + l^2 + l^2*tan(q2/2)^2 + xc1^2 + xc5^2 + xc1^2*tan(q2/2)^2 + xc5^2*tan(q2/2)^2 - 4*l*xc5*tan(q2/2) - 2*l*xc1*tan(q2/2)^2)*(2*l*xc1 - 3*l^2 - 3*l^2*tan(q2/2)^2 + xc1^2 + xc5^2 + xc1^2*tan(q2/2)^2 + xc5^2*tan(q2/2)^2 - 4*l*xc5*tan(q2/2) - 2*l*xc1*tan(q2/2)^2))^(1/2) - 4*l^2*tan(q2/2) + 2*l*xc5*tan(q2/2)^2)/(3*l^2*tan(q2/2)^2 - l^2 + xc1^2 + xc5^2 + xc1^2*tan(q2/2)^2 + xc5^2*tan(q2/2)^2 - 4*l*xc5*tan(q2/2) - 4*l*xc1*tan(q2/2)^2) - (4*(l*xc5 - 2*l^2*tan(q2/2) + l*xc5*tan(q2/2)^2))/(3*l^2*tan(q2/2)^2 - l^2 + xc1^2 + xc5^2 + xc1^2*tan(q2/2)^2 + xc5^2*tan(q2/2)^2 - 4*l*xc5*tan(q2/2) - 4*l*xc1*tan(q2/2)^2));
q4 = ...
2*atan((2*l*xc5 + (-(2*l*xc1 + l^2 + l^2*tan(q2/2)^2 + xc1^2 + xc5^2 + xc1^2*tan(q2/2)^2 + xc5^2*tan(q2/2)^2 - 4*l*xc5*tan(q2/2) - 2*l*xc1*tan(q2/2)^2)*(2*l*xc1 - 3*l^2 - 3*l^2*tan(q2/2)^2 + xc1^2 + xc5^2 + xc1^2*tan(q2/2)^2 + xc5^2*tan(q2/2)^2 - 4*l*xc5*tan(q2/2) - 2*l*xc1*tan(q2/2)^2))^(1/2) - 4*l^2*tan(q2/2) + 2*l*xc5*tan(q2/2)^2)/(3*l^2*tan(q2/2)^2 - l^2 + xc1^2 + xc5^2 + xc1^2*tan(q2/2)^2 + xc5^2*tan(q2/2)^2 - 4*l*xc5*tan(q2/2) - 4*l*xc1*tan(q2/2)^2)) + 2*atan((2*l*xc5 + (-(2*l*xc1 + l^2 + l^2*tan(q2/2)^2 + xc1^2 + xc5^2 + xc1^2*tan(q2/2)^2 + xc5^2*tan(q2/2)^2 - 4*l*xc5*tan(q2/2) - 2*l*xc1*tan(q2/2)^2)*(2*l*xc1 - 3*l^2 - 3*l^2*tan(q2/2)^2 + xc1^2 + xc5^2 + xc1^2*tan(q2/2)^2 + xc5^2*tan(q2/2)^2 - 4*l*xc5*tan(q2/2) - 2*l*xc1*tan(q2/2)^2))^(1/2) - 4*l^2*tan(q2/2) + 2*l*xc5*tan(q2/2)^2)/(3*l^2*tan(q2/2)^2 - l^2 + xc1^2 + xc5^2 + xc1^2*tan(q2/2)^2 + xc5^2*tan(q2/2)^2 - 4*l*xc5*tan(q2/2) - 4*l*xc1*tan(q2/2)^2) - (4*(l*xc5 - 2*l^2*tan(q2/2) + l*xc5*tan(q2/2)^2))/(3*l^2*tan(q2/2)^2 - l^2 + xc1^2 + xc5^2 + xc1^2*tan(q2/2)^2 + xc5^2*tan(q2/2)^2 - 4*l*xc5*tan(q2/2) - 4*l*xc1*tan(q2/2)^2));


I2 = ma*l^2/4 + 1/12 *ma*l^2;
I5 = I2;
I3 = I2 + 1/12 * ma*d^2 + ma*(d^2/4+l^2/4);

M =...
[      m1 + 2*ma,  0,                                        (I5*cos(q2 + q3) - I3*cos(q2 + q3 + q4))/(l*sin(q4)) - ma*(l*sin(q2 + q3) - 2*d*cos(q2 + q3) + 2*l*sin(q2));...
              0, m1,                                                                                              -(I5*sin(q2 + q3) - I3*sin(q2 + q3 + q4))/(l*sin(q4));...
-2*l*ma*sin(q2),  0, (I2*sin(q4) + I5*sin(q3) - I3*cos(q3)*sin(q4) - I3*cos(q4)*sin(q3) + 2*l^2*ma*sin(q4) + l^2*ma*cos(q3)*sin(q4) + 2*d*l*ma*sin(q3)*sin(q4))/sin(q4)];
 
tau=M*ddQ;
end

== matlab function controllo_giunti_2/robot ==
  data: tau input; Q output; Q_prev input; dQ_prev input; ddQ_prev input; ddq3_prev input; ddq4_prev input; dt input; parametri input; dQ output; ddQ output; Fex input
function [Q,dQ,ddQ] = robot(tau,Q_prev,dQ_prev,ddQ_prev,ddq3_prev,ddq4_prev,dt,parametri,Fex)%conosco tau e devo calcolare la velocità, è un problema di dinamica diretta
xc1=Q_prev(1);
xc5=Q_prev(2);
q2=Q_prev(3);

dxc1=dQ_prev(1);
dxc5=dQ_prev(2);
dq2=dQ_prev(3);

ddxc1=ddQ_prev(1);
ddxc5=ddQ_prev(2);
ddq2=ddQ_prev(3);

l=parametri(1);
d=parametri(2);
m1=parametri(3);
ma=parametri(4);
g=9.81;

Fx=Fex(1);
Fy=Fex(2);
Mf=Fex(3);

I2 = ma*l^2/4 + 1/12 *ma*l^2;
I5 = I2;
I3 = I2 + 1/12 * ma*d^2 + ma*(d^2/4+l^2/4);

q3 = ...
 -q2 - 2*atan((2*l*xc5 + (-(2*l*xc1 + l^2 + l^2*tan(q2/2)^2 + xc1^2 + xc5^2 + xc1^2*tan(q2/2)^2 + xc5^2*tan(q2/2)^2 - 4*l*xc5*tan(q2/2) - 2*l*xc1*tan(q2/2)^2)*(2*l*xc1 - 3*l^2 - 3*l^2*tan(q2/2)^2 + xc1^2 + xc5^2 + xc1^2*tan(q2/2)^2 + xc5^2*tan(q2/2)^2 - 4*l*xc5*tan(q2/2) - 2*l*xc1*tan(q2/2)^2))^(1/2) - 4*l^2*tan(q2/2) + 2*l*xc5*tan(q2/2)^2)/(3*l^2*tan(q2/2)^2 - l^2 + xc1^2 + xc5^2 + xc1^2*tan(q2/2)^2 + xc5^2*tan(q2/2)^2 - 4*l*xc5*tan(q2/2) - 4*l*xc1*tan(q2/2)^2) - (4*(l*xc5 - 2*l^2*tan(q2/2) + l*xc5*tan(q2/2)^2))/(3*l^2*tan(q2/2)^2 - l^2 + xc1^2 + xc5^2 + xc1^2*tan(q2/2)^2 + xc5^2*tan(q2/2)^2 - 4*l*xc5*tan(q2/2) - 4*l*xc1*tan(q2/2)^2));
q4 = ...
2*atan((2*l*xc5 + (-(2*l*xc1 + l^2 + l^2*tan(q2/2)^2 + xc1^2 + xc5^2 + xc1^2*tan(q2/2)^2 + xc5^2*tan(q2/2)^2 - 4*l*xc5*tan(q2/2) - 2*l*xc1*tan(q2/2)^2)*(2*l*xc1 - 3*l^2 - 3*l^2*tan(q2/2)^2 + xc1^2 + xc5^2 + xc1^2*tan(q2/2)^2 + xc5^2*tan(q2/2)^2 - 4*l*xc5*tan(q2/2) - 2*l*xc1*tan(q2/2)^2))^(1/2) - 4*l^2*tan(q2/2) + 2*l*xc5*tan(q2/2)^2)/(3*l^2*tan(q2/2)^2 - l^2 + xc1^2 + xc5^2 + xc1^2*tan(q2/2)^2 + xc5^2*tan(q2/2)^2 - 4*l*xc5*tan(q2/2) - 4*l*xc1*tan(q2/2)^2)) + 2*atan((2*l*xc5 + (-(2*l*xc1 + l^2 + l^2*tan(q2/2)^2 + xc1^2 + xc5^2 + xc1^2*tan(q2/2)^2 + xc5^2*tan(q2/2)^2 - 4*l*xc5*tan(q2/2) - 2*l*xc1*tan(q2/2)^2)*(2*l*xc1 - 3*l^2 - 3*l^2*tan(q2/2)^2 + xc1^2 + xc5^2 + xc1^2*tan(q2/2)^2 + xc5^2*tan(q2/2)^2 - 4*l*xc5*tan(q2/2) - 2*l*xc1*tan(q2/2)^2))^(1/2) - 4*l^2*tan(q2/2) + 2*l*xc5*tan(q2/2)^2)/(3*l^2*tan(q2/2)^2 - l^2 + xc1^2 + xc5^2 + xc1^2*tan(q2/2)^2 + xc5^2*tan(q2/2)^2 - 4*l*xc5*tan(q2/2) - 4*l*xc1*tan(q2/2)^2) - (4*(l*xc5 - 2*l^2*tan(q2/2) + l*xc5*tan(q2/2)^2))/(3*l^2*tan(q2/2)^2 - l^2 + xc1^2 + xc5^2 + xc1^2*tan(q2/2)^2 + xc5^2*tan(q2/2)^2 - 4*l*xc5*tan(q2/2) - 4*l*xc1*tan(q2/2)^2));

dq3 =...
(2*dxc5*((2*l + (4*sin(q2)*l^3 - 4*sin(2*q2)*l^2*xc1 - 4*cos(2*q2)*l^2*xc5 - 4*sin(q2)*l*xc1^2 + 8*cos(q2)*l*xc1*xc5 - 12*sin(q2)*l*xc5^2 + 4*xc1^2*xc5 + 4*xc5^3)/(2*(3*l^4 + 4*cos(q2)*l^3*xc1 - 4*sin(q2)*l^3*xc5 - 2*cos(2*q2)*l^2*xc1^2 + 4*sin(2*q2)*l^2*xc1*xc5 + 2*cos(2*q2)*l^2*xc5^2 - 4*cos(q2)*l*xc1^3 + 4*sin(q2)*l*xc1^2*xc5 - 4*cos(q2)*l*xc1*xc5^2 + 4*sin(q2)*l*xc5^3 - xc1^4 - 2*xc1^2*xc5^2 - xc5^4)^(1/2)))/(l^2 - 2*l*xc1 + xc1^2 + xc5^2 - 2*l^2*cos(q2) + 2*l*xc1*cos(q2) - 2*l*xc5*sin(q2)) + ((2*xc5 - 2*l*sin(q2))*(2*l^2*sin(q2) + (3*l^4 + 4*cos(q2)*l^3*xc1 - 4*sin(q2)*l^3*xc5 - 2*cos(2*q2)*l^2*xc1^2 + 4*sin(2*q2)*l^2*xc1*xc5 + 2*cos(2*q2)*l^2*xc5^2 - 4*cos(q2)*l*xc1^3 + 4*sin(q2)*l*xc1^2*xc5 - 4*cos(q2)*l*xc1*xc5^2 + 4*sin(q2)*l*xc5^3 - xc1^4 - 2*xc1^2*xc5^2 - xc5^4)^(1/2) - 2*l*xc5))/(l^2 - 2*l*xc1 + xc1^2 + xc5^2 - 2*l^2*cos(q2) + 2*l*xc1*cos(q2) - 2*l*xc5*sin(q2))^2))/((2*l^2*sin(q2) + (3*l^4 + 4*cos(q2)*l^3*xc1 - 4*sin(q2)*l^3*xc5 - 2*cos(2*q2)*l^2*xc1^2 + 4*sin(2*q2)*l^2*xc1*xc5 + 2*cos(2*q2)*l^2*xc5^2 - 4*cos(q2)*l*xc1^3 + 4*sin(q2)*l*xc1^2*xc5 - 4*cos(q2)*l*xc1*xc5^2 + 4*sin(q2)*l*xc5^3 - xc1^4 - 2*xc1^2*xc5^2 - xc5^4)^(1/2) - 2*l*xc5)^2/(l^2 - 2*l*xc1 + xc1^2 + xc5^2 - 2*l^2*cos(q2) + 2*l*xc1*cos(q2) - 2*l*xc5*sin(q2))^2 + 1) - dq2*((2*(((- 4*sin(q2)*l^3*xc1 - 4*cos(q2)*l^3*xc5 + 4*sin(2*q2)*l^2*xc1^2 + 8*cos(2*q2)*l^2*xc1*xc5 - 4*sin(2*q2)*l^2*xc5^2 + 4*sin(q2)*l*xc1^3 + 4*cos(q2)*l*xc1^2*xc5 + 4*sin(q2)*l*xc1*xc5^2 + 4*cos(q2)*l*xc5^3)/(2*(3*l^4 + 4*cos(q2)*l^3*xc1 - 4*sin(q2)*l^3*xc5 - 2*cos(2*q2)*l^2*xc1^2 + 4*sin(2*q2)*l^2*xc1*xc5 + 2*cos(2*q2)*l^2*xc5^2 - 4*cos(q2)*l*xc1^3 + 4*sin(q2)*l*xc1^2*xc5 - 4*cos(q2)*l*xc1*xc5^2 + 4*sin(q2)*l*xc5^3 - xc1^4 - 2*xc1^2*xc5^2 - xc5^4)^(1/2)) + 2*l^2*cos(q2))/(l^2 - 2*l*xc1 + xc1^2 + xc5^2 - 2*l^2*cos(q2) + 2*l*xc1*cos(q2) - 2*l*xc5*sin(q2)) + ((2*l*xc5*cos(q2) - 2*l^2*sin(q2) + 2*l*xc1*sin(q2))*(2*l^2*sin(q2) + (3*l^4 + 4*cos(q2)*l^3*xc1 - 4*sin(q2)*l^3*xc5 - 2*cos(2*q2)*l^2*xc1^2 + 4*sin(2*q2)*l^2*xc1*xc5 + 2*cos(2*q2)*l^2*xc5^2 - 4*cos(q2)*l*xc1^3 + 4*sin(q2)*l*xc1^2*xc5 - 4*cos(q2)*l*xc1*xc5^2 + 4*sin(q2)*l*xc5^3 - xc1^4 - 2*xc1^2*xc5^2 - xc5^4)^(1/2) - 2*l*xc5))/(l^2 - 2*l*xc1 + xc1^2 + xc5^2 - 2*l^2*cos(q2) + 2*l*xc1*cos(q2) - 2*l*xc5*sin(q2))^2))/((2*l^2*sin(q2) + (3*l^4 + 4*cos(q2)*l^3*xc1 - 4*sin(q2)*l^3*xc5 - 2*cos(2*q2)*l^2*xc1^2 + 4*sin(2*q2)*l^2*xc1*xc5 + 2*cos(2*q2)*l^2*xc5^2 - 4*cos(q2)*l*xc1^3 + 4*sin(q2)*l*xc1^2*xc5 - 4*cos(q2)*l*xc1*xc5^2 + 4*sin(q2)*l*xc5^3 - xc1^4 - 2*xc1^2*xc5^2 - xc5^4)^(1/2) - 2*l*xc5)^2/(l^2 - 2*l*xc1 + xc1^2 + xc5^2 - 2*l^2*cos(q2) + 2*l*xc1*cos(q2) - 2*l*xc5*sin(q2))^2 + 1) + 1) + (2*dxc1*(((2*xc1 - 2*l + 2*l*cos(q2))*(2*l^2*sin(q2) + (3*l^4 + 4*cos(q2)*l^3*xc1 - 4*sin(q2)*l^3*xc5 - 2*cos(2*q2)*l^2*xc1^2 + 4*sin(2*q2)*l^2*xc1*xc5 + 2*cos(2*q2)*l^2*xc5^2 - 4*cos(q2)*l*xc1^3 + 4*sin(q2)*l*xc1^2*xc5 - 4*cos(q2)*l*xc1*xc5^2 + 4*sin(q2)*l*xc5^3 - xc1^4 - 2*xc1^2*xc5^2 - xc5^4)^(1/2) - 2*l*xc5))/(l^2 - 2*l*xc1 + xc1^2 + xc5^2 - 2*l^2*cos(q2) + 2*l*xc1*cos(q2) - 2*l*xc5*sin(q2))^2 + (- 4*cos(q2)*l^3 + 4*cos(2*q2)*l^2*xc1 - 4*sin(2*q2)*l^2*xc5 + 12*cos(q2)*l*xc1^2 - 8*sin(q2)*l*xc1*xc5 + 4*cos(q2)*l*xc5^2 + 4*xc1^3 + 4*xc1*xc5^2)/(2*(l^2 - 2*l*xc1 + xc1^2 + xc5^2 - 2*l^2*cos(q2) + 2*l*xc1*cos(q2) - 2*l*xc5*sin(q2))*(3*l^4 + 4*cos(q2)*l^3*xc1 - 4*sin(q2)*l^3*xc5 - 2*cos(2*q2)*l^2*xc1^2 + 4*sin(2*q2)*l^2*xc1*xc5 + 2*cos(2*q2)*l^2*xc5^2 - 4*cos(q2)*l*xc1^3 + 4*sin(q2)*l*xc1^2*xc5 - 4*cos(q2)*l*xc1*xc5^2 + 4*sin(q2)*l*xc5^3 - xc1^4 - 2*xc1^2*xc5^2 - xc5^4)^(1/2))))/((2*l^2*sin(q2) + (3*l^4 + 4*cos(q2)*l^3*xc1 - 4*sin(q2)*l^3*xc5 - 2*cos(2*q2)*l^2*xc1^2 + 4*sin(2*q2)*l^2*xc1*xc5 + 2*cos(2*q2)*l^2*xc5^2 - 4*cos(q2)*l*xc1^3 + 4*sin(q2)*l*xc1^2*xc5 - 4*cos(q2)*l*xc1*xc5^2 + 4*sin(q2)*l*xc5^3 - xc1^4 - 2*xc1^2*xc5^2 - xc5^4)^(1/2) - 2*l*xc5)^2/(l^2 - 2*l*xc1 + xc1^2 + xc5^2 - 2*l^2*cos(q2) + 2*l*xc1*cos(q2) - 2*l*xc5*sin(q2))^2 + 1);

dq4 =...
 - dxc1*((2*(((2*xc1 - 2*l + 2*l*cos(q2))*((3*l^4 + 4*cos(q2)*l^3*xc1 - 4*sin(q2)*l^3*xc5 - 2*cos(2*q2)*l^2*xc1^2 + 4*sin(2*q2)*l^2*xc1*xc5 + 2*cos(2*q2)*l^2*xc5^2 - 4*cos(q2)*l*xc1^3 + 4*sin(q2)*l*xc1^2*xc5 - 4*cos(q2)*l*xc1*xc5^2 + 4*sin(q2)*l*xc5^3 - xc1^4 - 2*xc1^2*xc5^2 - xc5^4)^(1/2) - 2*l^2*sin(q2) + 2*l*xc5))/(l^2 - 2*l*xc1 + xc1^2 + xc5^2 - 2*l^2*cos(q2) + 2*l*xc1*cos(q2) - 2*l*xc5*sin(q2))^2 + (2*(xc1 + l*cos(q2))*(- l^2 + 2*cos(q2)*l*xc1 - 2*sin(q2)*l*xc5 + xc1^2 + xc5^2))/((l^2 - 2*l*xc1 + xc1^2 + xc5^2 - 2*l^2*cos(q2) + 2*l*xc1*cos(q2) - 2*l*xc5*sin(q2))*(3*l^4 + 4*cos(q2)*l^3*xc1 - 4*sin(q2)*l^3*xc5 - 2*cos(2*q2)*l^2*xc1^2 + 4*sin(2*q2)*l^2*xc1*xc5 + 2*cos(2*q2)*l^2*xc5^2 - 4*cos(q2)*l*xc1^3 + 4*sin(q2)*l*xc1^2*xc5 - 4*cos(q2)*l*xc1*xc5^2 + 4*sin(q2)*l*xc5^3 - xc1^4 - 2*xc1^2*xc5^2 - xc5^4)^(1/2))))/(((3*l^4 + 4*cos(q2)*l^3*xc1 - 4*sin(q2)*l^3*xc5 - 2*cos(2*q2)*l^2*xc1^2 + 4*sin(2*q2)*l^2*xc1*xc5 + 2*cos(2*q2)*l^2*xc5^2 - 4*cos(q2)*l*xc1^3 + 4*sin(q2)*l*xc1^2*xc5 - 4*cos(q2)*l*xc1*xc5^2 + 4*sin(q2)*l*xc5^3 - xc1^4 - 2*xc1^2*xc5^2 - xc5^4)^(1/2) - 2*l^2*sin(q2) + 2*l*xc5)^2/(l^2 - 2*l*xc1 + xc1^2 + xc5^2 - 2*l^2*cos(q2) + 2*l*xc1*cos(q2) - 2*l*xc5*sin(q2))^2 + 1) + (2*(((2*xc1 - 2*l + 2*l*cos(q2))*(2*l^2*sin(q2) + (3*l^4 + 4*cos(q2)*l^3*xc1 - 4*sin(q2)*l^3*xc5 - 2*cos(2*q2)*l^2*xc1^2 + 4*sin(2*q2)*l^2*xc1*xc5 + 2*cos(2*q2)*l^2*xc5^2 - 4*cos(q2)*l*xc1^3 + 4*sin(q2)*l*xc1^2*xc5 - 4*cos(q2)*l*xc1*xc5^2 + 4*sin(q2)*l*xc5^3 - xc1^4 - 2*xc1^2*xc5^2 - xc5^4)^(1/2) - 2*l*xc5))/(l^2 - 2*l*xc1 + xc1^2 + xc5^2 - 2*l^2*cos(q2) + 2*l*xc1*cos(q2) - 2*l*xc5*sin(q2))^2 + (2*(xc1 + l*cos(q2))*(- l^2 + 2*cos(q2)*l*xc1 - 2*sin(q2)*l*xc5 + xc1^2 + xc5^2))/((l^2 - 2*l*xc1 + xc1^2 + xc5^2 - 2*l^2*cos(q2) + 2*l*xc1*cos(q2) - 2*l*xc5*sin(q2))*(3*l^4 + 4*cos(q2)*l^3*xc1 - 4*sin(q2)*l^3*xc5 - 2*cos(2*q2)*l^2*xc1^2 + 4*sin(2*q2)*l^2*xc1*xc5 + 2*cos(2*q2)*l^2*xc5^2 - 4*cos(q2)*l*xc1^3 + 4*sin(q2)*l*xc1^2*xc5 - 4*cos(q2)*l*xc1*xc5^2 + 4*sin(q2)*l*xc5^3 - xc1^4 - 2*xc1^2*xc5^2 - xc5^4)^(1/2))))/((2*l^2*sin(q2) + (3*l^4 + 4*cos(q2)*l^3*xc1 - 4*sin(q2)*l^3*xc5 - 2*cos(2*q2)*l^2*xc1^2 + 4*sin(2*q2)*l^2*xc1*xc5 + 2*cos(2*q2)*l^2*xc5^2 - 4*cos(q2)*l*xc1^3 + 4*sin(q2)*l*xc1^2*xc5 - 4*cos(q2)*l*xc1*xc5^2 + 4*sin(q2)*l*xc5^3 - xc1^4 - 2*xc1^2*xc5^2 - xc5^4)^(1/2) - 2*l*xc5)^2/(l^2 - 2*l*xc1 + xc1^2 + xc5^2 - 2*l^2*cos(q2) + 2*l*xc1*cos(q2) - 2*l*xc5*sin(q2))^2 + 1)) - dxc5*((2*((2*l + (2*sin(q2)*l^3 - 2*sin(2*q2)*l^2*xc1 - 2*cos(2*q2)*l^2*xc5 - 2*sin(q2)*l*xc1^2 + 4*cos(q2)*l*xc1*xc5 - 6*sin(q2)*l*xc5^2 + 2*xc1^2*xc5 + 2*xc5^3)/(3*l^4 + 4*cos(q2)*l^3*xc1 - 4*sin(q2)*l^3*xc5 - 2*cos(2*q2)*l^2*xc1^2 + 4*sin(2*q2)*l^2*xc1*xc5 + 2*cos(2*q2)*l^2*xc5^2 - 4*cos(q2)*l*xc1^3 + 4*sin(q2)*l*xc1^2*xc5 - 4*cos(q2)*l*xc1*xc5^2 + 4*sin(q2)*l*xc5^3 - xc1^4 - 2*xc1^2*xc5^2 - xc5^4)^(1/2))/(l^2 - 2*l*xc1 + xc1^2 + xc5^2 - 2*l^2*cos(q2) + 2*l*xc1*cos(q2) - 2*l*xc5*sin(q2)) + ((2*xc5 - 2*l*sin(q2))*(2*l^2*sin(q2) + (3*l^4 + 4*cos(q2)*l^3*xc1 - 4*sin(q2)*l^3*xc5 - 2*cos(2*q2)*l^2*xc1^2 + 4*sin(2*q2)*l^2*xc1*xc5 + 2*cos(2*q2)*l^2*xc5^2 - 4*cos(q2)*l*xc1^3 + 4*sin(q2)*l*xc1^2*xc5 - 4*cos(q2)*l*xc1*xc5^2 + 4*sin(q2)*l*xc5^3 - xc1^4 - 2*xc1^2*xc5^2 - xc5^4)^(1/2) - 2*l*xc5))/(l^2 - 2*l*xc1 + xc1^2 + xc5^2 - 2*l^2*cos(q2) + 2*l*xc1*cos(q2) - 2*l*xc5*sin(q2))^2))/((2*l^2*sin(q2) + (3*l^4 + 4*cos(q2)*l^3*xc1 - 4*sin(q2)*l^3*xc5 - 2*cos(2*q2)*l^2*xc1^2 + 4*sin(2*q2)*l^2*xc1*xc5 + 2*cos(2*q2)*l^2*xc5^2 - 4*cos(q2)*l*xc1^3 + 4*sin(q2)*l*xc1^2*xc5 - 4*cos(q2)*l*xc1*xc5^2 + 4*sin(q2)*l*xc5^3 - xc1^4 - 2*xc1^2*xc5^2 - xc5^4)^(1/2) - 2*l*xc5)^2/(l^2 - 2*l*xc1 + xc1^2 + xc5^2 - 2*l^2*cos(q2) + 2*l*xc1*cos(q2) - 2*l*xc5*sin(q2))^2 + 1) - (2*((2*l - (2*sin(q2)*l^3 - 2*sin(2*q2)*l^2*xc1 - 2*cos(2*q2)*l^2*xc5 - 2*sin(q2)*l*xc1^2 + 4*cos(q2)*l*xc1*xc5 - 6*sin(q2)*l*xc5^2 + 2*xc1^2*xc5 + 2*xc5^3)/(3*l^4 + 4*cos(q2)*l^3*xc1 - 4*sin(q2)*l^3*xc5 - 2*cos(2*q2)*l^2*xc1^2 + 4*sin(2*q2)*l^2*xc1*xc5 + 2*cos(2*q2)*l^2*xc5^2 - 4*cos(q2)*l*xc1^3 + 4*sin(q2)*l*xc1^2*xc5 - 4*cos(q2)*l*xc1*xc5^2 + 4*sin(q2)*l*xc5^3 - xc1^4 - 2*xc1^2*xc5^2 - xc5^4)^(1/2))/(l^2 - 2*l*xc1 + xc1^2 + xc5^2 - 2*l^2*cos(q2) + 2*l*xc1*cos(q2) - 2*l*xc5*sin(q2)) - ((2*xc5 - 2*l*sin(q2))*((3*l^4 + 4*cos(q2)*l^3*xc1 - 4*sin(q2)*l^3*xc5 - 2*cos(2*q2)*l^2*xc1^2 + 4*sin(2*q2)*l^2*xc1*xc5 + 2*cos(2*q2)*l^2*xc5^2 - 4*cos(q2)*l*xc1^3 + 4*sin(q2)*l*xc1^2*xc5 - 4*cos(q2)*l*xc1*xc5^2 + 4*sin(q2)*l*xc5^3 - xc1^4 - 2*xc1^2*xc5^2 - xc5^4)^(1/2) - 2*l^2*sin(q2) + 2*l*xc5))/(l^2 - 2*l*xc1 + xc1^2 + xc5^2 - 2*l^2*cos(q2) + 2*l*xc1*cos(q2) - 2*l*xc5*sin(q2))^2))/(((3*l^4 + 4*cos(q2)*l^3*xc1 - 4*sin(q2)*l^3*xc5 - 2*cos(2*q2)*l^2*xc1^2 + 4*sin(2*q2)*l^2*xc1*xc5 + 2*cos(2*q2)*l^2*xc5^2 - 4*cos(q2)*l*xc1^3 + 4*sin(q2)*l*xc1^2*xc5 - 4*cos(q2)*l*xc1*xc5^2 + 4*sin(q2)*l*xc5^3 - xc1^4 - 2*xc1^2*xc5^2 - xc5^4)^(1/2) - 2*l^2*sin(q2) + 2*l*xc5)^2/(l^2 - 2*l*xc1 + xc1^2 + xc5^2 - 2*l^2*cos(q2) + 2*l*xc1*cos(q2) - 2*l*xc5*sin(q2))^2 + 1)) - dq2*((2*((2*l^2*cos(q2) - (2*l*(- sin(q2)*l^2*xc1 - cos(q2)*l^2*xc5 + sin(2*q2)*l*xc1^2 + 2*cos(2*q2)*l*xc1*xc5 - sin(2*q2)*l*xc5^2 + sin(q2)*xc1^3 + cos(q2)*xc1^2*xc5 + sin(q2)*xc1*xc5^2 + cos(q2)*xc5^3))/(3*l^4 + 4*cos(q2)*l^3*xc1 - 4*sin(q2)*l^3*xc5 - 2*cos(2*q2)*l^2*xc1^2 + 4*sin(2*q2)*l^2*xc1*xc5 + 2*cos(2*q2)*l^2*xc5^2 - 4*cos(q2)*l*xc1^3 + 4*sin(q2)*l*xc1^2*xc5 - 4*cos(q2)*l*xc1*xc5^2 + 4*sin(q2)*l*xc5^3 - xc1^4 - 2*xc1^2*xc5^2 - xc5^4)^(1/2))/(l^2 - 2*l*xc1 + xc1^2 + xc5^2 - 2*l^2*cos(q2) + 2*l*xc1*cos(q2) - 2*l*xc5*sin(q2)) - (2*l*(xc5*cos(q2) - l*sin(q2) + xc1*sin(q2))*((3*l^4 + 4*cos(q2)*l^3*xc1 - 4*sin(q2)*l^3*xc5 - 2*cos(2*q2)*l^2*xc1^2 + 4*sin(2*q2)*l^2*xc1*xc5 + 2*cos(2*q2)*l^2*xc5^2 - 4*cos(q2)*l*xc1^3 + 4*sin(q2)*l*xc1^2*xc5 - 4*cos(q2)*l*xc1*xc5^2 + 4*sin(q2)*l*xc5^3 - xc1^4 - 2*xc1^2*xc5^2 - xc5^4)^(1/2) - 2*l^2*sin(q2) + 2*l*xc5))/(l^2 - 2*l*xc1 + xc1^2 + xc5^2 - 2*l^2*cos(q2) + 2*l*xc1*cos(q2) - 2*l*xc5*sin(q2))^2))/(((3*l^4 + 4*cos(q2)*l^3*xc1 - 4*sin(q2)*l^3*xc5 - 2*cos(2*q2)*l^2*xc1^2 + 4*sin(2*q2)*l^2*xc1*xc5 + 2*cos(2*q2)*l^2*xc5^2 - 4*cos(q2)*l*xc1^3 + 4*sin(q2)*l*xc1^2*xc5 - 4*cos(q2)*l*xc1*xc5^2 + 4*sin(q2)*l*xc5^3 - xc1^4 - 2*xc1^2*xc5^2 - xc5^4)^(1/2) - 2*l^2*sin(q2) + 2*l*xc5)^2/(l^2 - 2*l*xc1 + xc1^2 + xc5^2 - 2*l^2*cos(q2) + 2*l*xc1*cos(q2) - 2*l*xc5*sin(q2))^2 + 1) - (2*((2*l^2*cos(q2) + (2*l*(- sin(q2)*l^2*xc1 - cos(q2)*l^2*xc5 + sin(2*q2)*l*xc1^2 + 2*cos(2*q2)*l*xc1*xc5 - sin(2*q2)*l*xc5^2 + sin(q2)*xc1^3 + cos(q2)*xc1^2*xc5 + sin(q2)*xc1*xc5^2 + cos(q2)*xc5^3))/(3*l^4 + 4*cos(q2)*l^3*xc1 - 4*sin(q2)*l^3*xc5 - 2*cos(2*q2)*l^2*xc1^2 + 4*sin(2*q2)*l^2*xc1*xc5 + 2*cos(2*q2)*l^2*xc5^2 - 4*cos(q2)*l*xc1^3 + 4*sin(q2)*l*xc1^2*xc5 - 4*cos(q2)*l*xc1*xc5^2 + 4*sin(q2)*l*xc5^3 - xc1^4 - 2*xc1^2*xc5^2 - xc5^4)^(1/2))/(l^2 - 2*l*xc1 + xc1^2 + xc5^2 - 2*l^2*cos(q2) + 2*l*xc1*cos(q2) - 2*l*xc5*sin(q2)) + (2*l*(xc5*cos(q2) - l*sin(q2) + xc1*sin(q2))*(2*l^2*sin(q2) + (3*l^4 + 4*cos(q2)*l^3*xc1 - 4*sin(q2)*l^3*xc5 - 2*cos(2*q2)*l^2*xc1^2 + 4*sin(2*q2)*l^2*xc1*xc5 + 2*cos(2*q2)*l^2*xc5^2 - 4*cos(q2)*l*xc1^3 + 4*sin(q2)*l*xc1^2*xc5 - 4*cos(q2)*l*xc1*xc5^2 + 4*sin(q2)*l*xc5^3 - xc1^4 - 2*xc1^2*xc5^2 - xc5^4)^(1/2) - 2*l*xc5))/(l^2 - 2*l*xc1 + xc1^2 + xc5^2 - 2*l^2*cos(q2) + 2*l*xc1*cos(q2) - 2*l*xc5*sin(q2))^2))/((2*l^2*sin(q2) + (3*l^4 + 4*cos(q2)*l^3*xc1 - 4*sin(q2)*l^3*xc5 - 2*cos(2*q2)*l^2*xc1^2 + 4*sin(2*q2)*l^2*xc1*xc5 + 2*cos(2*q2)*l^2*xc5^2 - 4*cos(q2)*l*xc1^3 + 4*sin(q2)*l*xc1^2*xc5 - 4*cos(q2)*l*xc1*xc5^2 + 4*sin(q2)*l*xc5^3 - xc1^4 - 2*xc1^2*xc5^2 - xc5^4)^(1/2) - 2*l*xc5)^2/(l^2 - 2*l*xc1 + xc1^2 + xc5^2 - 2*l^2*cos(q2) + 2*l*xc1*cos(q2) - 2*l*xc5*sin(q2))^2 + 1));

ddx2=ddxc1-l/2*(cos(q2)*dq2^2+sin(q2)*ddq2);
q5=q2+q3+q4-pi;
dq5=dq2+dq3+dq4;
ddq5=ddq2+ddq3_prev+ddq4_prev;
ddy4=ddxc5+ddq5*l/2*cos(q5)-dq5^2*l/2*sin(q5);

M =...
[      m1 + 2*ma,  0,                                        (I5*cos(q2 + q3) - I3*cos(q2 + q3 + q4))/(l*sin(q4)) - ma*(l*sin(q2 + q3) - 2*d*cos(q2 + q3) + 2*l*sin(q2));...
              0, m1,                                                                                              -(I5*sin(q2 + q3) - I3*sin(q2 + q3 + q4))/(l*sin(q4));...
-2*l*ma*sin(q2),  0, (I2*sin(q4) + I5*sin(q3) - I3*cos(q3)*sin(q4) - I3*cos(q4)*sin(q3) + 2*l^2*ma*sin(q4) + l^2*ma*cos(q3)*sin(q4) + 2*d*l*ma*sin(q3)*sin(q4))/sin(q4)];

G=...
[                  -(ma*(3*l*cos(q4) + 3*l*cos(2*q2 + 2*q3 + q4) - d*sin(q4) + d*sin(2*q2 + 2*q3 + q4)))/(4*l*sin(q4));...
(d*ma*cos(q4) - d*ma*cos(2*q2 + 2*q3 + q4) + 4*l*m1*sin(q4) + 5*l*ma*sin(q4) + 3*l*ma*sin(2*q2 + 2*q3 + q4))/(4*l*sin(q4));...
-(ma*(3*l*sin(q2 + 2*q3 + q4) - d*cos(q2 + 2*q3 + q4) - 6*l*sin(q2 + q4) + d*cos(q2 - q4) + 3*l*sin(q2 - q4)))/(4*sin(q4))];

V=...
   [(4*Mf*cos(q2 + q3 + q4) + 3*l*ma*cos(q4) + 3*l*ma*cos(2*q2 + 2*q3 + q4) - d*ma*sin(q4) + d*ma*sin(2*q2 + 2*q3 + q4) - 4*I3*ddq3_prev*cos(q2 + q3 + q4) + 4*I5*ddq3_prev*cos(q2 + q3) + 4*I5*ddq4_prev*cos(q2 + q3) - 4*Fx*l*sin(q4) - 4*dq2^2*l^2*ma*sin(q2 + q4) + 2*ddq3_prev*l^2*ma*cos(q2 + q3 + q4) + 4*dq2^2*l^2*ma*sin(q2 - q4) - 2*ddq3_prev*l^2*ma*cos(q2 + q3 - q4) - 3*g*l*ma*cos(q4) - 3*g*l*ma*cos(2*q2 + 2*q3 + q4) + d*g*ma*sin(q4) - d*g*ma*sin(2*q2 + 2*q3 + q4) + 4*ddx2*l*ma*sin(q4) - 2*dq2^2*l^2*ma*sin(q2 + q3 + q4) - 2*dq3^2*l^2*ma*sin(q2 + q3 + q4) + 2*dq2^2*l^2*ma*sin(q2 + q3 - q4) + 2*dq3^2*l^2*ma*sin(q2 + q3 - q4) + 4*d*ddq3_prev*l*ma*sin(q2 + q3 + q4) + 4*d*dq2^2*l*ma*cos(q2 + q3 + q4) + 4*d*dq3^2*l*ma*cos(q2 + q3 + q4) - 4*d*ddq3_prev*l*ma*sin(q2 + q3 - q4) - 4*dq2*dq3*l^2*ma*sin(q2 + q3 + q4) - 4*d*dq2^2*l*ma*cos(q2 + q3 - q4) - 4*d*dq3^2*l*ma*cos(q2 + q3 - q4) + 4*dq2*dq3*l^2*ma*sin(q2 + q3 - q4) + 8*d*dq2*dq3*l*ma*cos(q2 + q3 + q4) - 8*d*dq2*dq3*l*ma*cos(q2 + q3 - q4))/(4*l*sin(q4));...
                                                                                                                                                                                                                                                                                                                                                                                                                                                                                                                                                                                                                            -(4*Mf*sin(q2 + q3 + q4) + d*ma*cos(q4) - d*ma*cos(2*q2 + 2*q3 + q4) + 4*l*m1*sin(q4) + 5*l*ma*sin(q4) + 3*l*ma*sin(2*q2 + 2*q3 + q4) - 4*I3*ddq3_prev*sin(q2 + q3 + q4) + 4*I5*ddq3_prev*sin(q2 + q3) + 4*I5*ddq4_prev*sin(q2 + q3) - d*g*ma*cos(q4) + d*g*ma*cos(2*q2 + 2*q3 + q4) - 4*ddy4*l*ma*sin(q4) - 4*g*l*m1*sin(q4) - 5*g*l*ma*sin(q4) - 3*g*l*ma*sin(2*q2 + 2*q3 + q4))/(4*l*sin(q4));...
                                                       (4*Mf*sin(q3 + q4) + 2*Fx*l*cos(q2 - q4) + 2*Fy*l*sin(q2 - q4) + d*ma*cos(q2 - q4) + 3*l*ma*sin(q2 - q4) - d*ma*cos(q2 + 2*q3 + q4) - 2*Fx*l*cos(q2 + q4) + 3*l*ma*sin(q2 + 2*q3 + q4) - 4*I3*ddq3_prev*sin(q3 + q4) - 2*Fy*l*sin(q2 + q4) - 6*l*ma*sin(q2 + q4) + 4*I5*ddq3_prev*sin(q3) + 4*I5*ddq4_prev*sin(q3) + 2*dq2^2*l^2*ma*cos(q3 + q4) + 2*dq3^2*l^2*ma*cos(q3 + q4) + d*g*ma*cos(q2 + 2*q3 + q4) - 2*ddq3_prev*l^2*ma*sin(q3 - q4) - 3*g*l*ma*sin(q2 + 2*q3 + q4) + 6*g*l*ma*sin(q2 + q4) - 2*dq2^2*l^2*ma*cos(q3 - q4) - 2*dq3^2*l^2*ma*cos(q3 - q4) - d*g*ma*cos(q2 - q4) + 2*ddq3_prev*l^2*ma*sin(q3 + q4) - 3*g*l*ma*sin(q2 - q4) + 4*d*ddq3_prev*l*ma*cos(q3 - q4) + 4*dq2*dq3*l^2*ma*cos(q3 + q4) + 4*d*dq2^2*l*ma*sin(q3 + q4) + 4*d*dq3^2*l*ma*sin(q3 + q4) - 4*dq2*dq3*l^2*ma*cos(q3 - q4) - 4*d*dq2^2*l*ma*sin(q3 - q4) - 4*d*dq3^2*l*ma*sin(q3 - q4) - 4*d*ddq3_prev*l*ma*cos(q3 + q4) + 8*d*dq2*dq3*l*ma*sin(q3 + q4) - 8*d*dq2*dq3*l*ma*sin(q3 - q4))/(4*sin(q4))];


%ddq=inv(M)*(tau-N)  (N=V+G)
ddQ=M\(tau-V-G);
dQ=dQ_prev+ddQ*dt;
Q=Q_prev+dQ*dt;
end

== matlab function controllo_giunti_2/kin_dir1 ==
  data: Q input; P output; parametri input
function P  = kin_dir_pos(Q,parametri) %P[X Y alpha]
l=parametri(1);
d=parametri(2);
m1=parametri(3);
ma=parametri(4);
xc1=Q(1);
xc5=Q(2);
q2=Q(3);


q3 = ...
 -q2 - 2*atan((2*l*xc5 + (-(2*l*xc1 + l^2 + l^2*tan(q2/2)^2 + xc1^2 + xc5^2 + xc1^2*tan(q2/2)^2 + xc5^2*tan(q2/2)^2 - 4*l*xc5*tan(q2/2) - 2*l*xc1*tan(q2/2)^2)*(2*l*xc1 - 3*l^2 - 3*l^2*tan(q2/2)^2 + xc1^2 + xc5^2 + xc1^2*tan(q2/2)^2 + xc5^2*tan(q2/2)^2 - 4*l*xc5*tan(q2/2) - 2*l*xc1*tan(q2/2)^2))^(1/2) - 4*l^2*tan(q2/2) + 2*l*xc5*tan(q2/2)^2)/(3*l^2*tan(q2/2)^2 - l^2 + xc1^2 + xc5^2 + xc1^2*tan(q2/2)^2 + xc5^2*tan(q2/2)^2 - 4*l*xc5*tan(q2/2) - 4*l*xc1*tan(q2/2)^2) - (4*(l*xc5 - 2*l^2*tan(q2/2) + l*xc5*tan(q2/2)^2))/(3*l^2*tan(q2/2)^2 - l^2 + xc1^2 + xc5^2 + xc1^2*tan(q2/2)^2 + xc5^2*tan(q2/2)^2 - 4*l*xc5*tan(q2/2) - 4*l*xc1*tan(q2/2)^2));
q4 = ...
2*atan((2*l*xc5 + (-(2*l*xc1 + l^2 + l^2*tan(q2/2)^2 + xc1^2 + xc5^2 + xc1^2*tan(q2/2)^2 + xc5^2*tan(q2/2)^2 - 4*l*xc5*tan(q2/2) - 2*l*xc1*tan(q2/2)^2)*(2*l*xc1 - 3*l^2 - 3*l^2*tan(q2/2)^2 + xc1^2 + xc5^2 + xc1^2*tan(q2/2)^2 + xc5^2*tan(q2/2)^2 - 4*l*xc5*tan(q2/2) - 2*l*xc1*tan(q2/2)^2))^(1/2) - 4*l^2*tan(q2/2) + 2*l*xc5*tan(q2/2)^2)/(3*l^2*tan(q2/2)^2 - l^2 + xc1^2 + xc5^2 + xc1^2*tan(q2/2)^2 + xc5^2*tan(q2/2)^2 - 4*l*xc5*tan(q2/2) - 4*l*xc1*tan(q2/2)^2)) + 2*atan((2*l*xc5 + (-(2*l*xc1 + l^2 + l^2*tan(q2/2)^2 + xc1^2 + xc5^2 + xc1^2*tan(q2/2)^2 + xc5^2*tan(q2/2)^2 - 4*l*xc5*tan(q2/2) - 2*l*xc1*tan(q2/2)^2)*(2*l*xc1 - 3*l^2 - 3*l^2*tan(q2/2)^2 + xc1^2 + xc5^2 + xc1^2*tan(q2/2)^2 + xc5^2*tan(q2/2)^2 - 4*l*xc5*tan(q2/2) - 2*l*xc1*tan(q2/2)^2))^(1/2) - 4*l^2*tan(q2/2) + 2*l*xc5*tan(q2/2)^2)/(3*l^2*tan(q2/2)^2 - l^2 + xc1^2 + xc5^2 + xc1^2*tan(q2/2)^2 + xc5^2*tan(q2/2)^2 - 4*l*xc5*tan(q2/2) - 4*l*xc1*tan(q2/2)^2) - (4*(l*xc5 - 2*l^2*tan(q2/2) + l*xc5*tan(q2/2)^2))/(3*l^2*tan(q2/2)^2 - l^2 + xc1^2 + xc5^2 + xc1^2*tan(q2/2)^2 + xc5^2*tan(q2/2)^2 - 4*l*xc5*tan(q2/2) - 4*l*xc1*tan(q2/2)^2));


gamma = q2+q3;
%beta = q2+q3+q4;
alpha=gamma-pi/2;

P=zeros(3,1);
P(1) = xc1+l*cos(q2)+l/2*cos(gamma)+d*cos(alpha);
P(2) = l*sin(q2)+l/2*sin(gamma)+d*sin(alpha);
P(3) = q2 + q3 - pi/2;

end

== matlab function controllo_giunti_2/kin_dir2 ==
  data: Q input; P output; parametri input
function P  = kin_dir_pos(Q,parametri) %P[X Y alpha]
l=parametri(1);
d=parametri(2);
m1=parametri(3);
ma=parametri(4);
xc1=Q(1);
xc5=Q(2);
q2=Q(3);


q3 = ...
 -q2 - 2*atan((2*l*xc5 + (-(2*l*xc1 + l^2 + l^2*tan(q2/2)^2 + xc1^2 + xc5^2 + xc1^2*tan(q2/2)^2 + xc5^2*tan(q2/2)^2 - 4*l*xc5*tan(q2/2) - 2*l*xc1*tan(q2/2)^2)*(2*l*xc1 - 3*l^2 - 3*l^2*tan(q2/2)^2 + xc1^2 + xc5^2 + xc1^2*tan(q2/2)^2 + xc5^2*tan(q2/2)^2 - 4*l*xc5*tan(q2/2) - 2*l*xc1*tan(q2/2)^2))^(1/2) - 4*l^2*tan(q2/2) + 2*l*xc5*tan(q2/2)^2)/(3*l^2*tan(q2/2)^2 - l^2 + xc1^2 + xc5^2 + xc1^2*tan(q2/2)^2 + xc5^2*tan(q2/2)^2 - 4*l*xc5*tan(q2/2) - 4*l*xc1*tan(q2/2)^2) - (4*(l*xc5 - 2*l^2*tan(q2/2) + l*xc5*tan(q2/2)^2))/(3*l^2*tan(q2/2)^2 - l^2 + xc1^2 + xc5^2 + xc1^2*tan(q2/2)^2 + xc5^2*tan(q2/2)^2 - 4*l*xc5*tan(q2/2) - 4*l*xc1*tan(q2/2)^2));
q4 = ...
2*atan((2*l*xc5 + (-(2*l*xc1 + l^2 + l^2*tan(q2/2)^2 + xc1^2 + xc5^2 + xc1^2*tan(q2/2)^2 + xc5^2*tan(q2/2)^2 - 4*l*xc5*tan(q2/2) - 2*l*xc1*tan(q2/2)^2)*(2*l*xc1 - 3*l^2 - 3*l^2*tan(q2/2)^2 + xc1^2 + xc5^2 + xc1^2*tan(q2/2)^2 + xc5^2*tan(q2/2)^2 - 4*l*xc5*tan(q2/2) - 2*l*xc1*tan(q2/2)^2))^(1/2) - 4*l^2*tan(q2/2) + 2*l*xc5*tan(q2/2)^2)/(3*l^2*tan(q2/2)^2 - l^2 + xc1^2 + xc5^2 + xc1^2*tan(q2/2)^2 + xc5^2*tan(q2/2)^2 - 4*l*xc5*tan(q2/2) - 4*l*xc1*tan(q2/2)^2)) + 2*atan((2*l*xc5 + (-(2*l*xc1 + l^2 + l^2*tan(q2/2)^2 + xc1^2 + xc5^2 + xc1^2*tan(q2/2)^2 + xc5^2*tan(q2/2)^2 - 4*l*xc5*tan(q2/2) - 2*l*xc1*tan(q2/2)^2)*(2*l*xc1 - 3*l^2 - 3*l^2*tan(q2/2)^2 + xc1^2 + xc5^2 + xc1^2*tan(q2/2)^2 + xc5^2*tan(q2/2)^2 - 4*l*xc5*tan(q2/2) - 2*l*xc1*tan(q2/2)^2))^(1/2) - 4*l^2*tan(q2/2) + 2*l*xc5*tan(q2/2)^2)/(3*l^2*tan(q2/2)^2 - l^2 + xc1^2 + xc5^2 + xc1^2*tan(q2/2)^2 + xc5^2*tan(q2/2)^2 - 4*l*xc5*tan(q2/2) - 4*l*xc1*tan(q2/2)^2) - (4*(l*xc5 - 2*l^2*tan(q2/2) + l*xc5*tan(q2/2)^2))/(3*l^2*tan(q2/2)^2 - l^2 + xc1^2 + xc5^2 + xc1^2*tan(q2/2)^2 + xc5^2*tan(q2/2)^2 - 4*l*xc5*tan(q2/2) - 4*l*xc1*tan(q2/2)^2));


gamma = q2+q3;
%beta = q2+q3+q4;
alpha=gamma-pi/2;

P=zeros(3,1);
P(1) = xc1+l*cos(q2)+l/2*cos(gamma)+d*cos(alpha);
P(2) = l*sin(q2)+l/2*sin(gamma)+d*sin(alpha);
P(3) = q2 + q3 - pi/2;

end
